simulink model "SpringiLQR2discrete"  (R2021a)
settings: Solver=FixedStepDiscrete  StartTime=0.0  StopTime=100  FixedStep=0.001  MaxStep=0.01  RelTol=1e-3
undefined symbols (not defined in the file): A_e, Ad, B_e, Bd, C_e, Cd, D_e, Dd, Q, R, Su, Sx
libraries: pid_lib x1
settings Model: Creator=iris  LastModifiedBy=iris
settings SolverCC: AlgebraicLoopSolver=TrustRegion

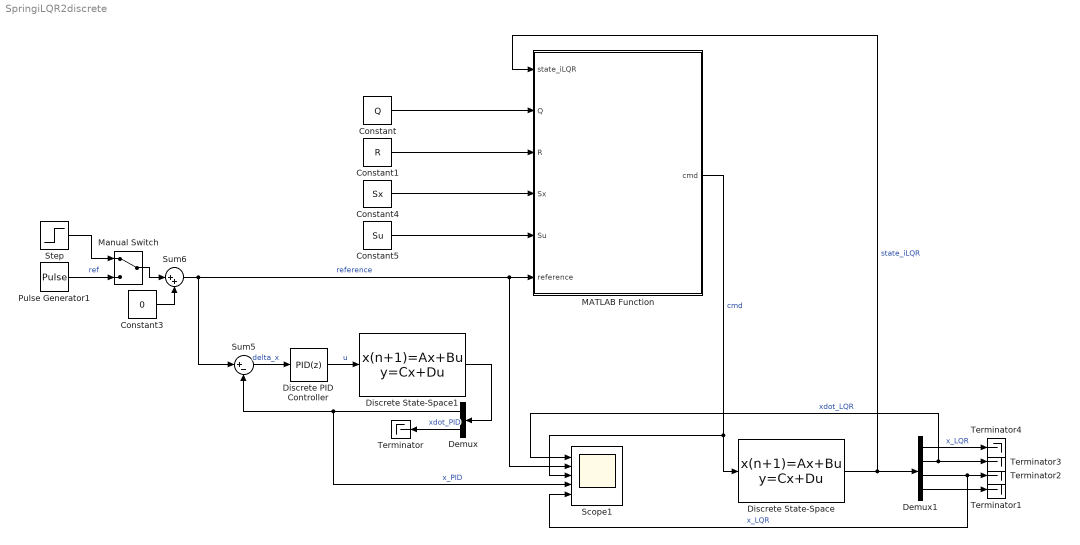
== system SpringiLQR2discrete ==
  Constant : Constant  Value=Q
  Constant1 : Constant  Value=R
  Constant3 : Constant  Value=0
  Constant4 : Constant  Value=Sx
  Constant5 : Constant  Value=Su
  Demux : Demux  Outputs=2
  Demux1 : Demux
  Discrete PID Controller : pid_lib/PID Controller  Controller=PID  Form=Parallel  TimeDomain=Discrete-time  UseExternalTs=off  SampleTime=-1  IntegratorMethod=Forward Euler  FilterMethod=Forward Euler  ControllerParametersSource=internal  P=8  I=4  D=3  UseFilter=on  N=100  TunerSelectOption=Transfer Function Based (PID Tuner App)  InitialConditionSource=internal  InitialConditionForIntegrator=0  InitialConditionForFilter=0  DifferentiatorICPrevScaledInput=0  ExternalReset=none  TrackingMode=off  Kt=1  LimitOutput=off  SatLimitsSource=internal  UpperSaturationLimit=inf  LowerSaturationLimit=-inf  LinearizeAsGain=off  AntiWindupMode=none  Kb=1  POutMin=[]  POutMax=[]  IOutMin=[]  IOutMax=[]  DOutMin=[]  DOutMax=[]  NOutMin=[]  NOutMax=[]  SumOutMin=[]  SumOutMax=[]  SaturationOutMin=[]  SaturationOutMax=[]  PParamMin=[]  PParamMax=[]  IParamMin=[]  IParamMax=[]  DParamMin=[]  DParamMax=[]  NParamMin=[]  NParamMax=[]  KbParamMin=[]  KbParamMax=[]  KtParamMin=[]  KtParamMax=[]  KbOutMin=[]  KbOutMax=[]  KtOutMin=[]  KtOutMax=[]  IntegratorOutMin=[]  IntegratorOutMax=[]  FilterOutMin=[]  FilterOutMax=[]  SumI1OutMin=[]  SumI1OutMax=[]  SumI2OutMin=[]  SumI2OutMax=[]  SumI3OutMin=[]  SumI3OutMax=[]  SumI4OutMin=[]  SumI4OutMax=[]  SumDOutMin=[]  SumDOutMax=[]  DifferentiatorOutMin=[]  DifferentiatorOutMax=[]  FilterDiffOutCoefMin=[]  FilterDiffOutCoefMax=[]  ReciprocalOutMin=[]  ReciprocalOutMax=[]  SumDenOutMin=[]  SumDenOutMax=[]  SumNumOutMin=[]  SumNumOutMax=[]  DivideOutMin=[]  DivideOutMax=[]  UdiffTsProdOutMin=[]  UdiffTsProdOutMax=[]  NTsProdOutMin=[]  NTsProdOutMax=[]  UintegralTsProdOutMin=[]  UintegralTsProdOutMax=[]  UngainTsProdOutMin=[]  UngainTsProdOutMax=[]  IntegratorContinuousStateAttributes=''  IntegratorStateMustResolveToSignalObject=off  IntegratorRTWStateStorageClass=Auto  FilterContinuousStateAttributes=''  FilterStateMustResolveToSignalObject=off  FilterRTWStateStorageClass=Auto  ParallelPVariant=InternalParameters  IdealPVariant=Disabled  IVariant=InternalParameters  DVariant=InternalParameters  IntegratorVariant=Discrete  SatVariant=Disabled  AWVariant=Passthrough  PCopyVariant=Disabled  TRVariant=Disabled  FdbkBlocksVariant=Forward  IdealPFdbkVariant=Disabled  SatFdbkVariant=Disabled  DerivativeFilterVariant=ForwardEulerFilter  NVariant=InternalParameters  NCopyVariant=Disabled  FilterICVariant=InternalICsFilter  IntegratorICVariant=InternalICs  ExternalResetVariant=Disabled  TRSumVariant=Passthrough  SumFdbkVariant=Disabled  SumVariant=Sum_PID  TsampFilterVariant=InternalTs  TsampNgainVariant=Passthrough  TsampIntegralVariant=Passthrough  ExternalSaturationOutDataTypeStr=Inherit: Same as second input
  Discrete State-Space : DiscreteStateSpace  A=A_e  B=B_e  C=C_e  D=D_e  SampleTime=-1
  Discrete State-Space1 : DiscreteStateSpace  A=Ad  B=Bd  C=Cd  D=Dd  SampleTime=-1
  MATLAB Function : MATLAB Function  TreatAsAtomicUnit=on
  Manual Switch : ManualSwitch
  Pulse Generator1 : DiscretePulseGenerator  PulseType=Time based  Period=20  PulseWidth=50
  Scope1 : Scope  NumInputPorts=5
  Step : Step  SampleTime=0
  Sum5 : Sum  Inputs=|+-
  Sum6 : Sum  Inputs=|++
  Terminator{,1..4} (5 alike) : Terminator
  wires:
  Pulse Generator1/1 -> Manual Switch/2  "ref"
  Discrete State-Space/1 -> MATLAB Function/1(state_iLQR), Demux1/1  "state_iLQR"
  Constant/1 -> MATLAB Function/2(Q)
  Constant1/1 -> MATLAB Function/3(R)
  MATLAB Function/1(cmd) -> Discrete State-Space/1, Scope1/3  "cmd"
  Sum5/1 -> Discrete PID Controller/1  "delta_x"
  Constant3/1 -> Sum6/2
  Sum6/1 -> Sum5/1, Scope1/2, MATLAB Function/6(reference)  "reference"
  Discrete PID Controller/1 -> Discrete State-Space1/1  "u"
  Discrete State-Space1/1 -> Demux/1
  Demux/1 -> Scope1/4, Sum5/2  "x_PID"
  Demux/2 -> Terminator/1  "xdot_PID"
  Constant4/1 -> MATLAB Function/4(Sx)
  Constant5/1 -> MATLAB Function/5(Su)
  Demux1/4 -> Terminator1/1
  Demux1/3 -> Scope1/5, Terminator2/1  "x_LQR"
  Demux1/1 -> Terminator4/1  "x_LQR"
  Demux1/2 -> Scope1/1, Terminator3/1  "xdot_LQR"
  Manual Switch/1 -> Sum6/1
  Step/1 -> Manual Switch/1

== matlab function SpringiLQR2discrete/MATLAB Function ==
  data: state_iLQR input; Q input; R input; Sx input; Su input; cmd output; reference input
function cmd = fcn(state_iLQR, Q, R,  Sx, Su, reference)



x_e = [state_iLQR];
Mu = ones(20,1)*reference;
cmd_e = (Su'*Q*Su+R)\Su'*Q*(Mu-Sx*x_e);
cmd = [cmd_e(1:2)];

end
